simulink model "simulink_discrete1Dy3D_Simulink"  (R2023b)
settings: Solver=ode45  StartTime=0.0  StopTime=0.7  RelTol=1e-3  EnableMultiTasking=on
values from neighbouring files (symbols this model uses):
  a1 = C_discrete.den{1,1}(2)    [control_float_test.m]
  a2 = C_discrete.den{1,1}(3)    [control_float_test.m]
  b0 = C_discrete.num{1,1}(1)    [control_float_test.m]
  b1 = C_discrete.num{1,1}(2)    [control_float_test.m]
  b2 = C_discrete.num{1,1}(3)    [control_float_test.m]
  T = T2    (= 0.001)    [control_float_test.m]
libraries: cstblocks x4
settings Model: Creator=Koldo  LastModifiedBy=chris
settings SolverCC: AlgebraicLoopSolver=TrustRegion
settings DataIOCC: LimitDataPoints=on  SaveFormat=Array  SignalLoggingSaveFormat=ModelDataLogs  ReturnWorkspaceOutputs=off
settings OptimizationCC: ExpressionDepthLimit=2147483647  LifeSpan=inf
settings DebuggingCC: UnderspecifiedInitializationDetection=Classic  MergeDetectMultiDrivingBlocksExec=none  SolverPrmCheckMsg=warning  FcnCallInpInsideContextMsg=warning  UnconnectedInputMsg=warning  UnconnectedOutputMsg=warning  UnconnectedLineMsg=warning  StateNameClashWarn=warning  SFUnexpectedBacktrackingDiag=warning  SFNoUnconditionalDefaultTransitionDiag=warning  SFExecutionAtInitializationDiag=none  ArithmeticOperatorsInVariantConditions=warning
settings HardwareCC: ProdBitPerPointer=32  ProdBitPerSizeT=32  ProdBitPerPtrDiffT=32  ProdLargestAtomicFloat=None  ProdIntDivRoundTo=Undefined  ProdEndianess=Unspecified  ProdWordSize=32  ProdHWDeviceType=32-bit Generic
settings ModelReferenceCC: EnableRefExpFcnMdlSchedulingChecks=on  PropagateSignalLabelsOutOfModel=off
settings SFSimCC: SimUseLocalCustomCode=off  CustomCodeUndefinedFunction=UseInterfaceOnly
settings RTWCC: RTWUseLocalCustomCode=off  DLArmComputeVersion=19.05
settings CodeAppCC: StateflowObjectComments=on
settings GRTTargetCC: TargetLangStandard=C89/C90 (ANSI)  CombineOutputUpdateFcns=off  GRTInterface=on
settings ConfigComp: CovMetricSettings=dw  CovSaveCumulativeToWorkspaceVar=on  CovSaveSingleToWorkspaceVar=on  CovExternalEMLEnable=off

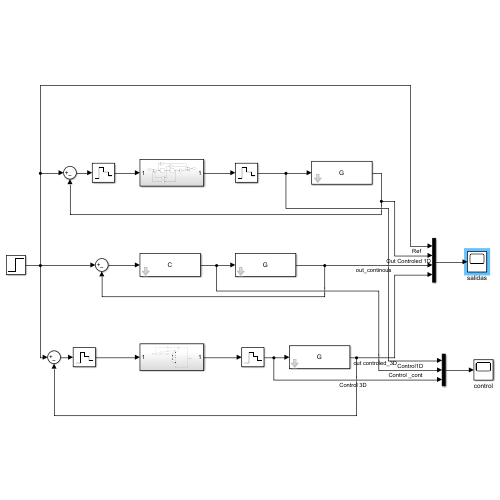
[thumbnail: Simulink's stored preview of the top-level diagram]
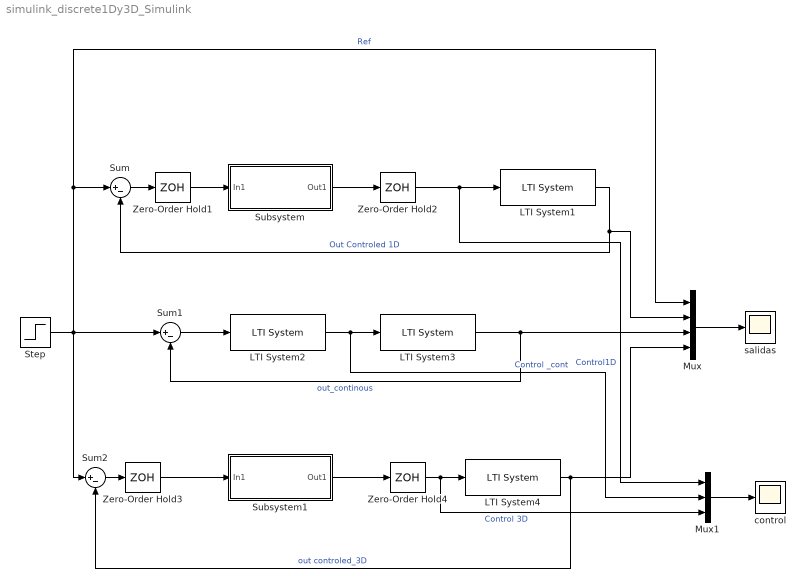
== system simulink_discrete1Dy3D_Simulink ==
  LTI System1 : cstblocks/LTI System  sys=G  IC=[]  PadeOrder=0
  LTI System2 : cstblocks/LTI System  sys=C  IC=[]  PadeOrder=0
  LTI System3 : cstblocks/LTI System  sys=G  IC=[]  PadeOrder=0
  LTI System4 : cstblocks/LTI System  sys=G  IC=[]  PadeOrder=0
  Mux : Mux
  Mux1 : Mux  Inputs=3
  Step : Step  Time=0  After=pi  SampleTime=0
  Subsystem : Subsystem
  Subsystem1 : Subsystem
  Sum : Sum  Inputs=|+-
  Sum1 : Sum  Inputs=|+-
  Sum2 : Sum  Inputs=|+-
  Zero-Order Hold{1..4} (4 alike) : ZeroOrderHold  SampleTime=T
  control : Scope
  salidas : Scope
  wires:
  Sum/1 -> Zero-Order Hold1/1
  LTI System1/1 -> Mux/2, Sum/2  "Out Controled 1D"
  Zero-Order Hold2/1 -> LTI System1/1, Mux1/1  "Control1D"
  Step/1 -> Sum2/1, Sum1/1, Sum/1, Mux/1  "Ref"
  Sum1/1 -> LTI System2/1
  LTI System3/1 -> Sum1/2, Mux/3  "out_continous"
  LTI System2/1 -> LTI System3/1, Mux1/2  "Control _cont"
  Mux/1 -> salidas/1
  Sum2/1 -> Zero-Order Hold3/1
  LTI System4/1 -> Mux/4, Sum2/2  "out controled_3D"
  Zero-Order Hold4/1 -> LTI System4/1, Mux1/3  "Control 3D"
  Mux1/1 -> control/1
  Subsystem1/1(Out1) -> Zero-Order Hold4/1
  Zero-Order Hold3/1 -> Subsystem1/1(In1)
  Subsystem/1(Out1) -> Zero-Order Hold2/1
  Zero-Order Hold1/1 -> Subsystem/1(In1)

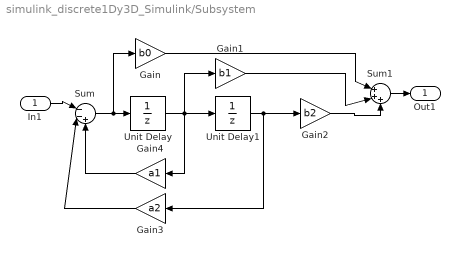
== system simulink_discrete1Dy3D_Simulink/Subsystem ==
  In1 : Inport
  Gain : Gain  Gain=b0
  Gain1 : Gain  Gain=b1
  Gain2 : Gain  Gain=b2
  Gain3 : Gain  Gain=a2
  Gain4 : Gain  Gain=a1
  Sum : Sum  Inputs=|--+
  Sum1 : Sum  Inputs=|+++
  Unit Delay : UnitDelay  SampleTime=-1  HasFrameUpgradeWarning=on
  Unit Delay1 : UnitDelay  SampleTime=-1  HasFrameUpgradeWarning=on
  Out1 : Outport
  wires:
  Sum1/1 -> Out1/1
  Unit Delay1/1 -> Gain2/1, Gain3/1
  Gain/1 -> Sum1/1
  Gain1/1 -> Sum1/2
  Gain2/1 -> Sum1/3
  Unit Delay/1 -> Unit Delay1/1, Gain4/1, Gain1/1
  Gain3/1 -> Sum/2
  Sum/1 -> Gain/1, Unit Delay/1
  Gain4/1 -> Sum/3
  In1/1 -> Sum/1

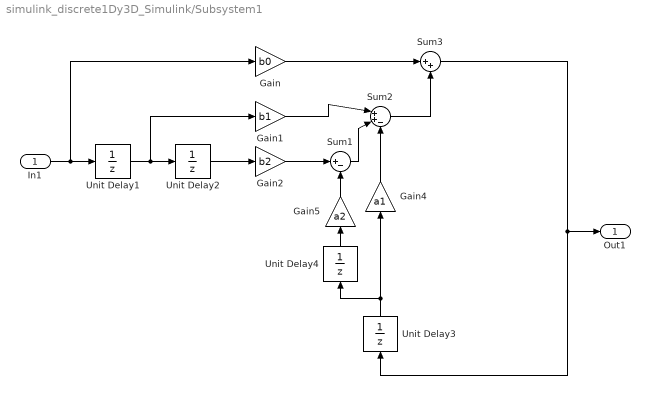
== system simulink_discrete1Dy3D_Simulink/Subsystem1 ==
  In1 : Inport
  Gain : Gain  Gain=b0
  Gain1 : Gain  Gain=b1
  Gain2 : Gain  Gain=b2
  Gain4 : Gain  Gain=a1
  Gain5 : Gain  Gain=a2
  Sum1 : Sum  Inputs=|+-
  Sum2 : Sum  Inputs=|++-
  Sum3 : Sum  Inputs=|++
  Unit Delay{1..4} (4 alike) : UnitDelay  SampleTime=-1  HasFrameUpgradeWarning=on
  Out1 : Outport
  wires:
  In1/1 -> Gain/1, Unit Delay1/1
  Unit Delay1/1 -> Gain1/1, Unit Delay2/1
  Unit Delay2/1 -> Gain2/1
  Gain2/1 -> Sum1/1
  Gain5/1 -> Sum1/2
  Gain1/1 -> Sum2/1
  Gain/1 -> Sum3/1
  Sum2/1 -> Sum3/2
  Gain4/1 -> Sum2/3
  Sum1/1 -> Sum2/2
  Sum3/1 -> Unit Delay3/1, Out1/1
  Unit Delay3/1 -> Unit Delay4/1, Gain4/1
  Unit Delay4/1 -> Gain5/1
